simulink model "simulate_copter"  (R2026a)
settings: Solver=ode4  StopTime=5
settings Model: Creator=Kiril  LastModifiedBy=User

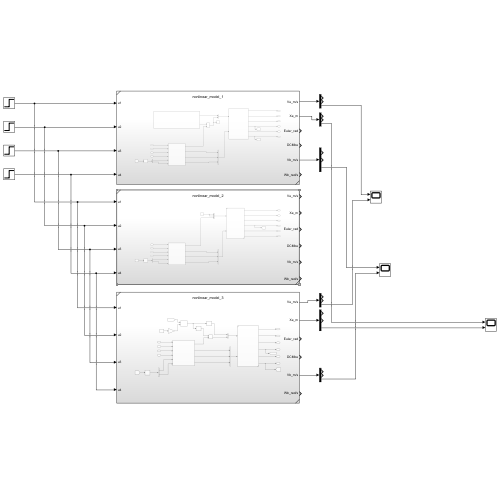
[thumbnail: Simulink's stored preview of the top-level diagram]
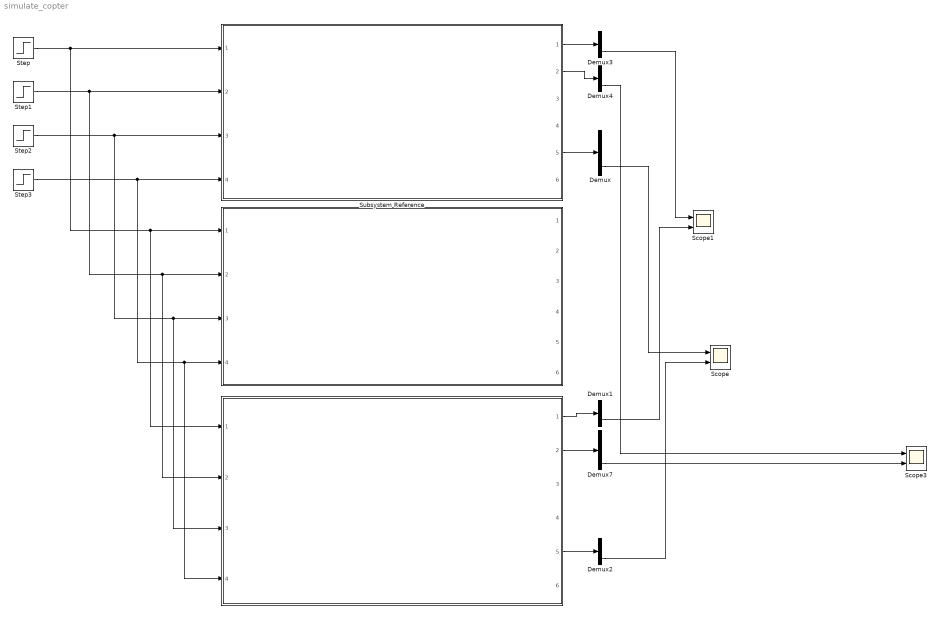
== system simulate_copter ==
  " " : Subsystem  ReferencedSubsystem=nonlinear_model_3
  "  " : Subsystem  ReferencedSubsystem=nonlinear_model_2
  Demux{,1..4,7} (6 alike) : Demux  Outputs=3
  Scope : Scope  NumInputPorts=2
      settings: ActiveDisplayYMinimum=-59.225581338911375  ActiveDisplayYMaximum=48.657306751783686
  Scope1 : Scope  NumInputPorts=2
      settings: ActiveDisplayYMinimum=-117.72566135734078  ActiveDisplayYMaximum=23.980629039704532
  Scope3 : Scope  NumInputPorts=2
      settings: ActiveDisplayYMinimum=-205.67422615420131  ActiveDisplayYMaximum=30.249706671283469  DataLoggingVariableName=ScopeData11
  Step : Step  FinalValue=1000  SampleTime=0
  Step1 : Step  FinalValue=1000  SampleTime=0
  Step2 : Step  FinalValue=1000  SampleTime=0
  Step3 : Step  FinalValue=500  SampleTime=0
  Subsystem Reference : Subsystem  ReferencedSubsystem=nonlinear_model_1
  wires:
  Subsystem Reference/5 -> Demux/1
  Demux/3 -> Scope/1
  Step/1 -> " "/1, "  "/1, Subsystem Reference/1
  Step1/1 -> " "/2, "  "/2, Subsystem Reference/2
  Step2/1 -> " "/3, "  "/3, Subsystem Reference/3
  Step3/1 -> " "/4, "  "/4, Subsystem Reference/4
  Subsystem Reference/1 -> Demux3/1
  Demux3/3 -> Scope1/1
  Subsystem Reference/2 -> Demux4/1
  Demux4/3 -> Scope3/1
  " "/2 -> Demux7/1
  Demux7/3 -> Scope3/2
  " "/1 -> Demux1/1
  Demux1/3 -> Scope1/2
  " "/5 -> Demux2/1
  Demux2/3 -> Scope/2
